simulink model "self_notworking"  (R2021b)
settings: Solver=VariableStepAuto  StartTime=0.0  StopTime=10.0  RelTol=1e-3

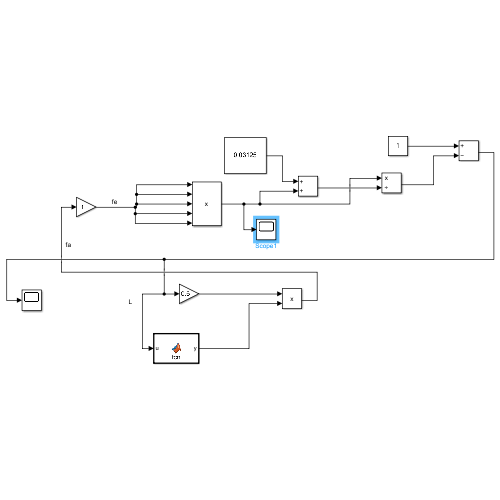
[thumbnail: Simulink's stored preview of the top-level diagram]
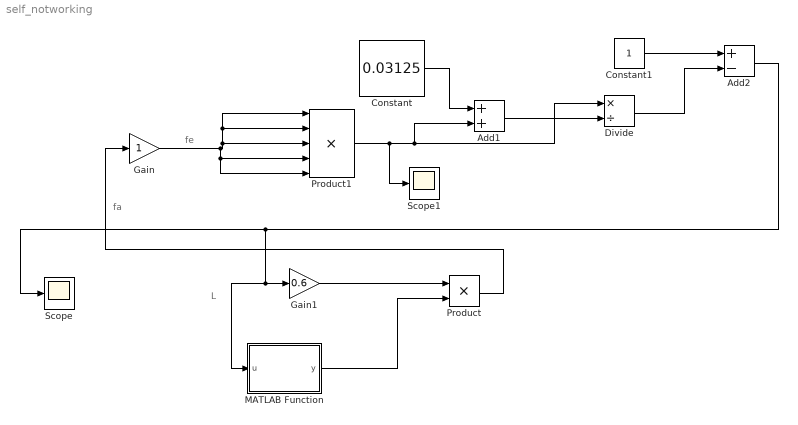
== system self_notworking ==
  note: fe
  note: fa
  note: L
  Add1 : Sum
  Add2 : Sum  Inputs=+-
  Constant : Constant  Value=0.03125
  Constant1 : Constant
  Divide : Product  Inputs=*/
  Gain : Gain
  Gain1 : Gain  Gain=0.6
  MATLAB Function : MATLAB Function  TreatAsAtomicUnit=on
  Product : Product
  Product1 : Product  Inputs=5
  Scope : Scope
  Scope1 : Scope
  wires:
  Gain1/1 -> Product/1
  MATLAB Function/1(y) -> Product/2
  Add2/1 -> Scope/1, MATLAB Function/1(u), Gain1/1
  Product/1 -> Gain/1
  Constant1/1 -> Add2/1
  Gain/1 -> Product1/5, Product1/4, Product1/3, Product1/2, Product1/1
  Product1/1 -> Scope1/1, Divide/1, Add1/2
  Constant/1 -> Add1/1
  Add1/1 -> Divide/2
  Divide/1 -> Add2/2

== matlab function self_notworking/MATLAB Function ==
  data: u input; y output
function y = fcn(u)

y = (exp(0.5*u));
